simulink model "AMCLIB_FW_BAM"  (Simulink 9.3)
settings: Solver=VariableStepAuto  StartTime=0.0  StopTime=10.0  RelTol=1e-3
settings Model: Creator=nxa18952  LastModifiedBy=nxa18952
settings DataIOCC: SaveFormat=Dataset  SignalLoggingSaveFormat=Dataset  ReturnWorkspaceOutputs=on
settings OptimizationCC: LifeSpan=auto
settings DebuggingCC: UnderspecifiedInitializationDetection=Simplified  MergeDetectMultiDrivingBlocksExec=error  FcnCallInpInsideContextMsg=error  SFUnexpectedBacktrackingDiag=error  SFNoUnconditionalDefaultTransitionDiag=error  SFExecutionAtInitializationDiag=warning  ArithmeticOperatorsInVariantConditions=error
settings HardwareCC: ProdBitPerPointer=64  ProdBitPerSizeT=64  ProdBitPerPtrDiffT=64  ProdLargestAtomicFloat=Float  ProdIntDivRoundTo=Zero  ProdEndianess=LittleEndian  ProdWordSize=64  ProdHWDeviceType=Intel->x86-64 (Windows64)
settings ModelReferenceCC: PropagateSignalLabelsOutOfModel=on
settings SFSimCC: SimUseLocalCustomCode=on
settings RTWCC: RTWUseLocalCustomCode=on
settings CodeAppCC: StateflowObjectComments=off
settings GRTTargetCC: TargetLangStandard=C99 (ISO)  CombineOutputUpdateFcns=on  GRTInterface=off
settings ConfigComp: CovMetricSettings=dwe  CovHtmlReporting=off  CovSaveCumulativeToWorkspaceVar=off  CovSaveSingleToWorkspaceVar=off  CovExternalEMLEnable=on

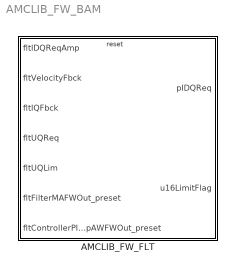
== system AMCLIB_FW_BAM ==
  AMCLIB_FW_FLT : Subsystem  TreatAsAtomicUnit=on  mask(AMCLIB_FW_FLT){showStates=Hide (faster execution), resetStatesEnable=Pre-set according to the first set of inputs after reset, showDebugOutputs=Hide, fltUmaxDivImax=0, fltLambda=0, fltPropGain=0, fltIntegGain=0, fltLowerLimit=0, fltUpperLimit=0}
      mask prompts: showStates "Show internal states"; resetStatesEnable "Internal state after reset"; showDebugOutputs "Show debugging outputs"; fltUmaxDivImax "fltUmaxDivImax (Maximal coil voltage divided by the maximal coil current)"; fltLambda "fltLambda (GDFLIB_FilterMA - smoothing factor)"; fltPropGain "fltPropGain (GFLIB_ControllerPIpAW - proportional gain)"; fltIntegGain "fltIntegGain (GFLIB_ControllerPIpAW - integral gain)"; fltLowerLimit "fltLowerLimit (GFLIB_ControllerPIpAW - lower limit)"; fltUpperLimit "fltUpperLimit (GFLIB_ControllerPIpAW - upper limit)"
      mask help: Field Weakening controller for the PMSM field-oriented control algorithm in single precision floating-point implementation. This block supports re-initialization of the internal state during simulation. If the block is reset, the output of the MA filter and PI controller will be aligned with the inputs fltFilterMAFWOut_preset and fltControllerPIpAWFWOut_preset. Refer to the AMMCLIB User's Guide for further details.
      mask init:
      | if ~evalin('base','exist(''tS8'',''var'')')
      |   if (2 ~= exist('SWLIBS_Typedefs.mat','file'))
      |       error('File SWLIBS_Typedefs.mat is not on the Matlab path. Please add the AMMCLIB "bam" folder in the Matlab Search Path.');
      |   else
      |       evalin('base', 'load(''SWLIBS_Typedefs.mat'')');
      |   end
      | end
      | if showStates == 1
      |     % hidden state variables
      |     if strcmp(get_param([gcb '/fltUmaxDivImax'], 'BlockType'), 'Inport')
      |         posblk = get_param(gcb, 'Position');
      | 
      |         pos = get_param(    [gcb, '/fltUmaxDivImax'], 'Position');
      |         orient = get_param( [gcb, '/fltUmaxDivImax'], 'Orientation');
      |         delete_block(       [gcb, '/fltUmaxDivImax']);
      |         add_block('built-in/Ground', [gcb, '/fltUmaxDivImax'], 'Position', pos, 'Orientation', orient);
      | 
      |         pos = get_param(    [gcb, '/fltLambda'], 'Position');
      |         orient = get_param( [gcb, '/fltLambda'], 'Orientation');
      |         delete_block(       [gcb, '/fltLambda']);
      |         add_block('built-in/Ground', [gcb, '/fltLambda'], 'Position', pos, 'Orientation', orient);
      | 
      |         pos = get_param(    [gcb, '/fltPropGain'], 'Position');
      |         orient = get_param( [gcb, '/fltPropGain'], 'Orientation');
      |         delete_block(       [gcb, '/fltPropGain']);
      |         add_block('built-in/Ground', [gcb, '/fltPropGain'], 'Position', pos, 'Orientation', orient);
      | 
      |         pos = get_param(    [gcb, '/fltIntegGain'], 'Position');
      |         orient = get_param( [gcb, '/fltIntegGain'], 'Orientation');
      |         delete_block(       [gcb, '/fltIntegGain']);
      |         add_block('built-in/Ground', [gcb, '/fltIntegGain'], 'Position', pos, 'Orientation', orient);
      | 
      |         pos = get_param(    [gcb, '/fltLowerLimit'], 'Position');
      |         orient = get_param( [gcb, '/fltLowerLimit'], 'Orientation');
      |         delete_block(       [gcb, '/fltLowerLimit']);
      |         add_block('built-in/Ground', [gcb, '/fltLowerLimit'], 'Position', pos, 'Orientation', orient);
      | 
      |         pos = get_param(    [gcb, '/fltUpperLimit'], 'Position');
      |         orient = get_param( [gcb, '/fltUpperLimit'], 'Orientation');
      |         delete_block(       [gcb, '/fltUpperLimit']);
      |         add_block('built-in/Ground', [gcb, '/fltUpperLimit'], 'Position', pos, 'Orientation', orient);
      | 
      |         pos = get_param(    [gcb, '/fltIQReqK_1'], 'Position');
      |         orient = get_param( [gcb, '/fltIQReqK_1'], 'Orientation');
      |         delete_block(       [gcb, '/fltIQReqK_1']);
      |         add_block('built-in/Ground', [gcb, '/fltIQReqK_1'], 'Position', pos, 'Orientation', orient);
      | 
      |         pos = get_param(    [gcb, '/fltAcc'], 'Position');
      |         orient = get_param( [gcb, '/fltAcc'], 'Orientation');
      |         delete_block(       [gcb, '/fltAcc']);
      |         add_block('built-in/Ground', [gcb, '/fltAcc'], 'Position', pos, 'Orientation', orient);
      | 
      |         pos = get_param(    [gcb, '/fltIntegPartK_1'], 'Position');
      |         orient = get_param( [gcb, '/fltIntegPartK_1'], 'Orientation');
      |         delete_block(       [gcb, '/fltIntegPartK_1']);
      |         add_block('built-in/Ground', [gcb, '/fltIntegPartK_1'], 'Position', pos, 'Orientation', orient);
      | 
      |         pos = get_param(    [gcb, '/fltInK_1'], 'Position');
      |         orient = get_param( [gcb, '/fltInK_1'], 'Orientation');
      |         delete_block(       [gcb, '/fltInK_1']);
      |         add_block('built-in/Ground', [gcb, '/fltInK_1'], 'Position', pos, 'Orientation', orient);
      | 
      | 
      |         pos = get_param(    [gcb '/fltAcc_Out'], 'Position');
      |         orient = get_param( [gcb '/fltAcc_Out'], 'Orientation');
      |         delete_block(       [gcb '/fltAcc_Out']);
      |         add_block('built-in/Terminator', [gcb '/fltAcc_Out'], 'Position', pos, 'Orientation', orient);
      | 
      |         pos = get_param(    [gcb '/fltIntegPartK_1_Out'], 'Position');
      |         orient = get_param( [gcb '/fltIntegPartK_1_Out'], 'Orientation');
      |         delete_block(       [gcb '/fltIntegPartK_1_Out']);
      |         add_block('built-in/Terminator', [gcb '/fltIntegPartK_1_Out'], 'Position', pos, 'Orientation', orient);
      | 
      |         pos = get_param(    [gcb '/fltInK_1_Out'], 'Position');
      |         orient = get_param( [gcb '/fltInK_1_Out'], 'Orientation');
      |         delete_block(       [gcb '/fltInK_1_Out']);
      |         add_block('built-in/Terminator', [gcb '/fltInK_1_Out'], 'Position', pos, 'Orientation', orient);
      | 
      | 
      |         if strcmp(get_param([gcb '/fltIQErrSign'], 'BlockType'), 'Outport')
      |             pos = get_param(    [gcb '/fltIQErrSign'], 'Position');
      |             orient = get_param( [gcb '/fltIQErrSign'], 'Orientation');
      |             delete_block(       [gcb '/fltIQErrSign']);
      |             add_block('built-in/Terminator', [gcb '/fltIQErrSign'], 'Position', pos, 'Orientation', orient);
      | 
      |             pos = get_param(    [gcb '/fltIQErr'], 'Position');
      |             orient = get_param( [gcb '/fltIQErr'], 'Orientation');
      |             delete_block(       [gcb '/fltIQErr']);
      |             add_block('built-in/Terminator', [gcb '/fltIQErr'], 'Position', pos, 'Orientation', orient);
      | 
      |             pos = get_param(    [gcb '/fltFWErr'], 'Position');
      |             orient = get_param( [gcb '/fltFWErr'], 'Orientation');
      |             delete_block(       [gcb '/fltFWErr']);
      |             add_block('built-in/Terminator', [gcb '/fltFWErr'], 'Position', pos, 'Orientation', orient);
      | 
      |             pos = get_param(    [gcb '/fltUQErr'], 'Position');
      |             orient = get_param( [gcb '/fltUQErr'], 'Orientation');
      |             delete_block(       [gcb '/fltUQErr']);
      |             add_block('built-in/Terminator', [gcb '/fltUQErr'], 'Position', pos, 'Orientation', orient);
      | 
      |             pos = get_param(    [gcb '/fltFWErrFilt'], 'Position');
      |             orient = get_param( [gcb '/fltFWErrFilt'], 'Orientation');
      |             delete_block(       [gcb '/fltFWErrFilt']);
      |             add_block('built-in/Terminator', [gcb '/fltFWErrFilt'], 'Position', pos, 'Orientation', orient);
      | 
      |             pos = get_param(    [gcb '/fltFWAngle'], 'Position');
      |             orient = get_param( [gcb '/fltFWAngle'], 'Orientation');
      |             delete_block(       [gcb '/fltFWAngle']);
      |             add_block('built-in/Terminator', [gcb '/fltFWAngle'], 'Position', pos, 'Orientation', orient);
      | 
      |             pos = get_param(    [gcb '/fltFWSin'], 'Position');
      |             orient = get_param( [gcb '/fltFWSin'], 'Orientation');
      |             delete_block(       [gcb '/fltFWSin']);
      |             add_block('built-in/Terminator', [gcb '/fltFWSin'], 'Position', pos, 'Orientation', orient);
      | 
      |             pos = get_param(    [gcb '/fltFWCos'], 'Position');
      |             orient = get_param( [gcb '/fltFWCos'], 'Orientation');
      |             delete_block(       [gcb '/fltFWCos']);
      |             add_block('built-in/Terminator', [gcb '/fltFWCos'], 'Position', pos, 'Orientation', orient);
      | 
      |         end
      | 
      |         set_param([gcb '/fltIDQReqAmp'], 'Port', '1');
      |         set_param([gcb '/fltVelocityFbck'], 'Port', '2');
      |         set_param([gcb '/fltIQFbck'], 'Port', '3');
      |         set_param([gcb '/fltUQReq'], 'Port', '4');
      |         set_param([gcb '/fltUQLim'], 'Port', '5');
      |         set_param([gcb '/fltFilterMAFWOut_preset'], 'Port', '6');
      |         set_param([gcb '/fltControllerPIpAWFWOut_preset'], 'Port', '7');
      | 
      |         set_param([gcb '/pIDQReq'], 'Port', '1');
      |         set_param([gcb '/u16LimitFlag'], 'Port', '2');
      | 
      |         set_param(gcb,'MaskEnables',{'on','on','off','on','on','on','on','on','on'});
      | 
      |         if (posblk(4) - posblk(2)) > 200
      |           height = 200;
      |           set_param(gcb,'Position',[posblk(1), posblk(2), posblk(3), posblk(2)+height])
      |         end
      |     end
      | else
      |     % shown state variables
      |     if strcmp(get_param([gcb '/fltUmaxDivImax'], 'BlockType'), 'Ground')
      |         posblk = get_param(gcb, 'Position');
      | 
      |         pos = get_param(    [gcb, '/fltUmaxDivImax'], 'Position');
      |         orient = get_param( [gcb, '/fltUmaxDivImax'], 'Orientation');
      |         delete_block(       [gcb, '/fltUmaxDivImax']);
      |         add_block('built-in/Inport', [gcb, '/fltUmaxDivImax'], 'Position', pos, 'Orientation', orient, 'OutDataTypeStr', 'single');
      | 
      |         pos = get_param(    [gcb, '/fltLambda'], 'Position');
      |         orient = get_param( [gcb, '/fltLambda'], 'Orientation');
      |         delete_block(       [gcb, '/fltLambda']);
      |         add_block('built-in/Inport', [gcb, '/fltLambda'], 'Position', pos, 'Orientation', orient, 'OutDataTypeStr', 'single');
      | 
      |         pos = get_param(    [gcb, '/fltPropGain'], 'Position');
      |         orient = get_param( [gcb, '/fltPropGain'], 'Orientation');
      |         delete_block(       [gcb, '/fltPropGain']);
      |         add_block('built-in/Inport', [gcb, '/fltPropGain'], 'Position', pos, 'Orientation', orient, 'OutDataTypeStr', 'single');
      | 
      |         pos = get_param(    [gcb, '/fltIntegGain'], 'Position');
      |         orient = get_param( [gcb, '/fltIntegGain'], 'Orientation');
      |         delete_block(       [gcb, '/fltIntegGain']);
      |         add_block('built-in/Inport', [gcb, '/fltIntegGain'], 'Position', pos, 'Orientation', orient, 'OutDataTypeStr', 'single');
      | 
      |         pos = get_param(    [gcb, '/fltLowerLimit'], 'Position');
      |         orient = get_param( [gcb, '/fltLowerLimit'], 'Orientation');
      |         delete_block(       [gcb, '/fltLowerLimit']);
      |         add_block('built-in/Inport', [gcb, '/fltLowerLimit'], 'Position', pos, 'Orientation', orient, 'OutDataTypeStr', 'single');
      | 
      |         pos = get_param(    [gcb, '/fltUpperLimit'], 'Position');
      |         orient = get_param( [gcb, '/fltUpperLimit'], 'Orientation');
      |         delete_block(       [gcb, '/fltUpperLimit']);
      |         add_block('built-in/Inport', [gcb, '/fltUpperLimit'], 'Position', pos, 'Orientation', orient, 'OutDataTypeStr', 'single');
      | 
      |         pos = get_param(    [gcb, '/fltIQReqK_1'], 'Position');
      |         orient = get_param( [gcb, '/fltIQReqK_1'], 'Orientation');
      |         delete_block(       [gcb, '/fltIQReqK_1']);
      |         add_block('built-in/Inport', [gcb, '/fltIQReqK_1'], 'Position', pos, 'Orientation', orient, 'OutDataTypeStr', 'single');
      | 
      |         pos = get_param(    [gcb, '/fltAcc'], 'Position');
      |         orient = get_param( [gcb, '/fltAcc'], 'Orientation');
      |         delete_block(       [gcb, '/fltAcc']);
      |         add_block('built-in/Inport', [gcb, '/fltAcc'], 'Position', pos, 'Orientation', orient, 'OutDataTypeStr', 'single');
      | 
      |         pos = get_param(    [gcb, '/fltIntegPartK_1'], 'Position');
      |         orient = get_param( [gcb, '/fltIntegPartK_1'], 'Orientation');
      |         delete_block(       [gcb, '/fltIntegPartK_1']);
      |         add_block('built-in/Inport', [gcb, '/fltIntegPartK_1'], 'Position', pos, 'Orientation', orient, 'OutDataTypeStr', 'single');
      | 
      |         pos = get_param(    [gcb, '/fltInK_1'], 'Position');
      |         orient = get_param( [gcb, '/fltInK_1'], 'Orientation');
      |         delete_block(       [gcb, '/fltInK_1']);
      |         add_block('built-in/Inport', [gcb, '/fltInK_1'], 'Position', pos, 'Orientation', orient, 'OutDataTypeStr', 'single');
      | 
      | 
      |         pos = get_param(    [gcb '/fltAcc_Out'], 'Position');
      |         orient = get_param( [gcb '/fltAcc_Out'], 'Orientation');
      |         delete_block(       [gcb '/fltAcc_Out']);
      |         add_block('built-in/Outport', [gcb '/fltAcc_Out'], 'Position', pos, 'Orientation', orient);
      | 
      |         pos = get_param(    [gcb '/fltIntegPartK_1_Out'], 'Position');
      |         orient = get_param( [gcb '/fltIntegPartK_1_Out'], 'Orientation');
      |         delete_block(       [gcb '/fltIntegPartK_1_Out']);
      |         add_block('built-in/Outport', [gcb '/fltIntegPartK_1_Out'], 'Position', pos, 'Orientation', orient);
      | 
      |         pos = get_param(    [gcb '/fltInK_1_Out'], 'Position');
      |         orient = get_param( [gcb '/fltInK_1_Out'], 'Orientation');
      |         delete_block(       [gcb '/fltInK_1_Out']);
      |         add_block('built-in/Outport', [gcb '/fltInK_1_Out'], 'Position', pos, 'Orientation', orient);
      | 
      | 
      |         if (showDebugOutputs == 2) && (strcmp(get_param([gcb '/fltIQErrSign'], 'BlockType'), 'Terminator'))
      |             pos = get_param(    [gcb '/fltIQErrSign'], 'Position');
      |             orient = get_param( [gcb '/fltIQErrSign'], 'Orientation');
      |             delete_block(       [gcb '/fltIQErrSign']);
      |             add_block('built-in/Outport', [gcb '/fltIQErrSign'], 'Position', pos, 'Orientation', orient);
      | 
      |             pos = get_param(    [gcb '/fltIQErr'], 'Position');
      |             orient = get_param( [gcb '/fltIQErr'], 'Orientation');
      |             delete_block(       [gcb '/fltIQErr']);
      |             add_block('built-in/Outport', [gcb '/fltIQErr'], 'Position', pos, 'Orientation', orient);
      | 
      |             pos = get_param(    [gcb '/fltFWErr'], 'Position');
      |             orient = get_param( [gcb '/fltFWErr'], 'Orientation');
      |             delete_block(       [gcb '/fltFWErr']);
      |             add_block('built-in/Outport', [gcb '/fltFWErr'], 'Position', pos, 'Orientation', orient);
      | 
      |             pos = get_param(    [gcb '/fltUQErr'], 'Position');
      |             orient = get_param( [gcb '/fltUQErr'], 'Orientation');
      |             delete_block(       [gcb '/fltUQErr']);
      |             add_block('built-in/Outport', [gcb '/fltUQErr'], 'Position', pos, 'Orientation', orient);
      | 
      |             pos = get_param(    [gcb '/fltFWErrFilt'], 'Position');
      |             orient = get_param( [gcb '/fltFWErrFilt'], 'Orientation');
      |             delete_block(       [gcb '/fltFWErrFilt']);
      |             add_block('built-in/Outport', [gcb '/fltFWErrFilt'], 'Position', pos, 'Orientation', orient);
      | 
      |             pos = get_param(    [gcb '/fltFWAngle'], 'Position');
      |             orient = get_param( [gcb '/fltFWAngle'], 'Orientation');
      |             delete_block(       [gcb '/fltFWAngle']);
      |             add_block('built-in/Outport', [gcb '/fltFWAngle'], 'Position', pos, 'Orientation', orient);
      | 
      |             pos = get_param(    [gcb '/fltFWSin'], 'Position');
      |             orient = get_param( [gcb '/fltFWSin'], 'Orientation');
      |             delete_block(       [gcb '/fltFWSin']);
      |             add_block('built-in/Outport', [gcb '/fltFWSin'], 'Position', pos, 'Orientation', orient);
      | 
      |             pos = get_param(    [gcb '/fltFWCos'], 'Position');
      |             orient = get_param( [gcb '/fltFWCos'], 'Orientation');
      |             delete_block(       [gcb '/fltFWCos']);
      |             add_block('built-in/Outport', [gcb '/fltFWCos'], 'Position', pos, 'Orientation', orient);
      | 
      |         end
      | 
      |         set_param([gcb '/fltIDQReqAmp'], 'Port', '1');
      |         set_param([gcb '/fltVelocityFbck'], 'Port', '2');
      |         set_param([gcb '/fltIQFbck'], 'Port', '3');
      |         set_param([gcb '/fltUQReq'], 'Port', '4');
      |         set_param([gcb '/fltUQLim'], 'Port', '5');
      |         set_param([gcb '/fltFilterMAFWOut_preset'], 'Port', '6');
      |         set_param([gcb '/fltControllerPIpAWFWOut_preset'], 'Port', '7');
      |         set_param([gcb '/fltUmaxDivImax'], 'Port', '8');
      |         set_param([gcb '/fltLambda'], 'Port', '9');
      |         set_param([gcb '/fltPropGain'], 'Port', '10');
      |         set_param([gcb '/fltIntegGain'], 'Port', '11');
      |         set_param([gcb '/fltLowerLimit'], 'Port', '12');
      |         set_param([gcb '/fltUpperLimit'], 'Port', '13');
      |         set_param([gcb '/fltIQReqK_1'], 'Port', '14');
      |         set_param([gcb '/fltAcc'], 'Port', '15');
      |         set_param([gcb '/fltIntegPartK_1'], 'Port', '16');
      |         set_param([gcb '/fltInK_1'], 'Port', '17');
      | 
      |         if (showDebugOutputs == 2)
      |             set_param([gcb '/pIDQReq'], 'Port', '1');
      |             set_param([gcb '/u16LimitFlag'], 'Port', '2');
      |             set_param([gcb '/fltIQErrSign'], 'Port', '3');
      |             set_param([gcb '/fltIQErr'], 'Port', '4');
      |             set_param([gcb '/fltFWErr'], 'Port', '5');
      |             set_param([gcb '/fltUQErr'], 'Port', '6');
      |             set_param([gcb '/fltFWErrFilt'], 'Port', '7');
      |             set_param([gcb '/fltFWAngle'], 'Port', '8');
      |             set_param([gcb '/fltFWSin'], 'Port', '9');
      |             set_param([gcb '/fltFWCos'], 'Port', '10');
      |             set_param([gcb '/fltAcc_Out'], 'Port', '11');
      |             set_param([gcb '/fltIntegPartK_1_Out'], 'Port', '12');
      |             set_param([gcb '/fltInK_1_Out'], 'Port', '13');
      |         else
      |             set_param([gcb '/pIDQReq'], 'Port', '1');
      |             set_param([gcb '/u16LimitFlag'], 'Port', '2');
      |             set_param([gcb '/fltAcc_Out'], 'Port', '3');
      |             set_param([gcb '/fltIntegPartK_1_Out'], 'Port', '4');
      |             set_param([gcb '/fltInK_1_Out'], 'Port', '5');
      |         end
      | 
      |         set_param(gcb,'MaskEnables',{'on','on','on','off','off','off','off','off','off'});
      | 
      |         if (posblk(4) - posblk(2)) < 450
      |           height = 450;
      |           set_param(gcb,'Position',[posblk(1), posblk(2), posblk(3), posblk(2)+height])
      |         end
      |     else
      |         if (showDebugOutputs == 2) && (strcmp(get_param([gcb '/fltIQErrSign'], 'BlockType'), 'Terminator'))
      |             % shown debugging outputs
      |             pos = get_param(    [gcb '/fltIQErrSign'], 'Position');
      |             orient = get_param( [gcb '/fltIQErrSign'], 'Orientation');
      |             delete_block(       [gcb '/fltIQErrSign']);
      |             add_block('built-in/Outport', [gcb '/fltIQErrSign'], 'Position', pos, 'Orientation', orient);
      | 
      |             pos = get_param(    [gcb '/fltIQErr'], 'Position');
      |             orient = get_param( [gcb '/fltIQErr'], 'Orientation');
      |             delete_block(       [gcb '/fltIQErr']);
      |             add_block('built-in/Outport', [gcb '/fltIQErr'], 'Position', pos, 'Orientation', orient);
      | 
      |             pos = get_param(    [gcb '/fltFWErr'], 'Position');
      |             orient = get_param( [gcb '/fltFWErr'], 'Orientation');
      |             delete_block(       [gcb '/fltFWErr']);
      |             add_block('built-in/Outport', [gcb '/fltFWErr'], 'Position', pos, 'Orientation', orient);
      | 
      |             pos = get_param(    [gcb '/fltUQErr'], 'Position');
      |             orient = get_param( [gcb '/fltUQErr'], 'Orientation');
      |             delete_block(       [gcb '/fltUQErr']);
      |             add_block('built-in/Outport', [gcb '/fltUQErr'], 'Position', pos, 'Orientation', orient);
      | 
      |             pos = get_param(    [gcb '/fltFWErrFilt'], 'Position');
      |             orient = get_param( [gcb '/fltFWErrFilt'], 'Orientation');
      |             delete_block(       [gcb '/fltFWErrFilt']);
      |             add_block('built-in/Outport', [gcb '/fltFWErrFilt'], 'Position', pos, 'Orientation', orient);
      | 
      |             pos = get_param(    [gcb '/fltFWAngle'], 'Position');
      |             orient = get_param( [gcb '/fltFWAngle'], 'Orientation');
      |             delete_block(       [gcb '/fltFWAngle']);
      |             add_block('built-in/Outport', [gcb '/fltFWAngle'], 'Position', pos, 'Orientation', orient);
      | 
      |             pos = get_param(    [gcb '/fltFWSin'], 'Position');
      |             orient = get_param( [gcb '/fltFWSin'], 'Orientation');
      |             delete_block(       [gcb '/fltFWSin']);
      |             add_block('built-in/Outport', [gcb '/fltFWSin'], 'Position', pos, 'Orientation', orient);
      | 
      |             pos = get_param(    [gcb '/fltFWCos'], 'Position');
      |             orient = get_param( [gcb '/fltFWCos'], 'Orientation');
      |             delete_block(       [gcb '/fltFWCos']);
      |             add_block('built-in/Outport', [gcb '/fltFWCos'], 'Position', pos, 'Orientation', orient);
      | 
      |             set_param([gcb '/pIDQReq'], 'Port', '1');
      |             set_param([gcb '/u16LimitFlag'], 'Port', '2');
      |             set_param([gcb '/fltIQErrSign'], 'Port', '3');
      |             set_param([gcb '/fltIQErr'], 'Port', '4');
      |             set_param([gcb '/fltFWErr'], 'Port', '5');
      |             set_param([gcb '/fltUQErr'], 'Port', '6');
      |             set_param([gcb '/fltFWErrFilt'], 'Port', '7');
      |             set_param([gcb '/fltFWAngle'], 'Port', '8');
      |             set_param([gcb '/fltFWSin'], 'Port', '9');
      |             set_param([gcb '/fltFWCos'], 'Port', '10');
      |             set_param([gcb '/fltAcc_Out'], 'Port', '11');
      |             set_param([gcb '/fltIntegPartK_1_Out'], 'Port', '12');
      |             set_param([gcb '/fltInK_1_Out'], 'Port', '13');
      |         elseif (showDebugOutputs == 1) && (strcmp(get_param([gcb '/fltIQErrSign'], 'BlockType'), 'Outport'))
      |             % hidden debugging outputs
      |             pos = get_param(    [gcb '/fltIQErrSign'], 'Position');
      |             orient = get_param( [gcb '/fltIQErrSign'], 'Orientation');
      |             delete_block(       [gcb '/fltIQErrSign']);
      |             add_block('built-in/Terminator', [gcb '/fltIQErrSign'], 'Position', pos, 'Orientation', orient);
      | 
      |             pos = get_param(    [gcb '/fltIQErr'], 'Position');
      |             orient = get_param( [gcb '/fltIQErr'], 'Orientation');
      |             delete_block(       [gcb '/fltIQErr']);
      |             add_block('built-in/Terminator', [gcb '/fltIQErr'], 'Position', pos, 'Orientation', orient);
      | 
      |             pos = get_param(    [gcb '/fltFWErr'], 'Position');
      |             orient = get_param( [gcb '/fltFWErr'], 'Orientation');
      |             delete_block(       [gcb '/fltFWErr']);
      |             add_block('built-in/Terminator', [gcb '/fltFWErr'], 'Position', pos, 'Orientation', orient);
      | 
      |             pos = get_param(    [gcb '/fltUQErr'], 'Position');
      |             orient = get_param( [gcb '/fltUQErr'], 'Orientation');
      |             delete_block(       [gcb '/fltUQErr']);
      |             add_block('built-in/Terminator', [gcb '/fltUQErr'], 'Position', pos, 'Orientation', orient);
      | 
      |             pos = get_param(    [gcb '/fltFWErrFilt'], 'Position');
      |             orient = get_param( [gcb '/fltFWErrFilt'], 'Orientation');
      |             delete_block(       [gcb '/fltFWErrFilt']);
      |             add_block('built-in/Terminator', [gcb '/fltFWErrFilt'], 'Position', pos, 'Orientation', orient);
      | 
      |             pos = get_param(    [gcb '/fltFWAngle'], 'Position');
      |             orient = get_param( [gcb '/fltFWAngle'], 'Orientation');
      |             delete_block(       [gcb '/fltFWAngle']);
      |             add_block('built-in/Terminator', [gcb '/fltFWAngle'], 'Position', pos, 'Orientation', orient);
      | 
      |             pos = get_param(    [gcb '/fltFWSin'], 'Position');
      |             orient = get_param( [gcb '/fltFWSin'], 'Orientation');
      |             delete_block(       [gcb '/fltFWSin']);
      |             add_block('built-in/Terminator', [gcb '/fltFWSin'], 'Position', pos, 'Orientation', orient);
      | 
      |             pos = get_param(    [gcb '/fltFWCos'], 'Position');
      |             orient = get_param( [gcb '/fltFWCos'], 'Orientation');
      |             delete_block(       [gcb '/fltFWCos']);
      |             add_block('built-in/Terminator', [gcb '/fltFWCos'], 'Position', pos, 'Orientation', orient);
      | 
      |             set_param([gcb '/pIDQReq'], 'Port', '1');
      |             set_param([gcb '/u16LimitFlag'], 'Port', '2');
      |             set_param([gcb '/fltAcc_Out'], 'Port', '3');
      |             set_param([gcb '/fltIntegPartK_1_Out'], 'Port', '4');
      |             set_param([gcb '/fltInK_1_Out'], 'Port', '5');
      |         end
      |     end
      | end
      settings: RTWSystemCode=Inline
      mask TypeOptions showStates: Hide (faster execution) | Show (allows debugging; connect feedback loops manually)
      mask Callback showStates:
      | maskStr = get_param(gcb,'showStates');
      | if strcmp(maskStr,'Hide (faster execution)'),
      |     set_param(gcb,'MaskEnables',{'on','on','off','on','on','on','on','on','on'});
      | else
      |     set_param(gcb,'MaskEnables',{'on','on','on','off','off','off','off','off','off'});
      | end
      mask TypeOptions resetStatesEnable: Pre-set according to the first set of inputs after reset | Clear to zero
      mask TypeOptions showDebugOutputs: Hide | Show
      mask Display:
      | color('black');
      | pos = get_param(gcb, 'Position');
      | width = pos(3) - pos(1);
      | height = pos(4) - pos(2);
      | tX=width/2;
      | tY=height - 25;
      | color('black');
      | text(tX,tY, 'AMCLIB_FW_FLT', 'horizontalAlignment', 'center');
      | if showStates == 2
      |   color('red');
      |   text(tX,tY - 20, ['debugging mode' char(13) char(10) '(limited performance)'], 'horizontalAlignment', 'center');
      | end

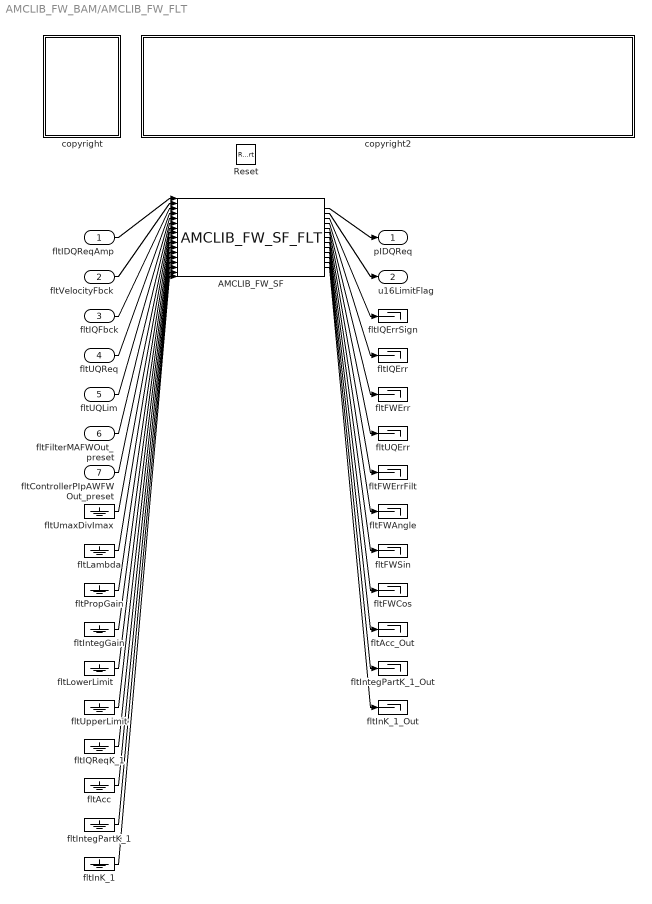
== system AMCLIB_FW_BAM/AMCLIB_FW_FLT ==
  fltIDQReqAmp : Inport  OutDataTypeStr=single
  fltVelocityFbck : Inport  Port=2  OutDataTypeStr=single
  fltIQFbck : Inport  Port=3  OutDataTypeStr=single
  fltUQReq : Inport  Port=4  OutDataTypeStr=single
  fltUQLim : Inport  Port=5  OutDataTypeStr=single
  fltFilterMAFWOut_preset : Inport  Port=6  OutDataTypeStr=single
  fltControllerPIpAWFWOut_preset : Inport  Port=7  OutDataTypeStr=single
  Reset : ResetPort  DisableCoverage=on
  AMCLIB_FW_SF : S-Function  FunctionName=AMCLIB_FW_SF_FLT  Parameters=showStates,resetStatesEnable,showDebugOutputs,fltUmaxDivImax,fltLambda,fltPropGain,fltIntegGain,fltLowerLimit,fltUpperLimit  SFunctionDeploymentMode=off  EnableBusSupport=off
  copyright : Subsystem
      mask Display: text(10,90,'FILE:');text(10,75,'DESRIPTION:');text(10,60,'COPYRIGHT:');text(10,45,'VERSION:');text(10,30,'DATE:')
  copyright2 : Subsystem
      mask Display: text(10,90,'AMCLIB_FW_BAM_FLT.mdl');text(10,75,'PMSM Field Weakening Controller');text(10,60,'NXP 2020');text(10,45,'1.0');text(10,30,'28-Mar-2020');
  fltAcc : Ground
  fltAcc_Out : Terminator
  fltFWAngle : Terminator
  fltFWCos : Terminator
  fltFWErr : Terminator
  fltFWErrFilt : Terminator
  fltFWSin : Terminator
  fltIQErr : Terminator
  fltIQErrSign : Terminator
  fltIQReqK_1 : Ground
  fltInK_1 : Ground
  fltInK_1_Out : Terminator
  fltIntegGain : Ground
  fltIntegPartK_1 : Ground
  fltIntegPartK_1_Out : Terminator
  fltLambda : Ground
  fltLowerLimit : Ground
  fltPropGain : Ground
  fltUQErr : Terminator
  fltUmaxDivImax : Ground
  fltUpperLimit : Ground
  pIDQReq : Outport
  u16LimitFlag : Outport  Port=2
  wires:
  fltIDQReqAmp/1 -> AMCLIB_FW_SF/1
  fltVelocityFbck/1 -> AMCLIB_FW_SF/2
  fltIQFbck/1 -> AMCLIB_FW_SF/3
  fltUQReq/1 -> AMCLIB_FW_SF/4
  fltUQLim/1 -> AMCLIB_FW_SF/5
  fltFilterMAFWOut_preset/1 -> AMCLIB_FW_SF/6
  fltControllerPIpAWFWOut_preset/1 -> AMCLIB_FW_SF/7
  fltUmaxDivImax/1 -> AMCLIB_FW_SF/8
  fltLambda/1 -> AMCLIB_FW_SF/9
  fltPropGain/1 -> AMCLIB_FW_SF/10
  fltIntegGain/1 -> AMCLIB_FW_SF/11
  fltLowerLimit/1 -> AMCLIB_FW_SF/12
  fltUpperLimit/1 -> AMCLIB_FW_SF/13
  fltIQReqK_1/1 -> AMCLIB_FW_SF/14
  fltAcc/1 -> AMCLIB_FW_SF/15
  fltIntegPartK_1/1 -> AMCLIB_FW_SF/16
  fltInK_1/1 -> AMCLIB_FW_SF/17
  AMCLIB_FW_SF/1 -> pIDQReq/1
  AMCLIB_FW_SF/2 -> u16LimitFlag/1
  AMCLIB_FW_SF/3 -> fltIQErrSign/1
  AMCLIB_FW_SF/4 -> fltIQErr/1
  AMCLIB_FW_SF/5 -> fltFWErr/1
  AMCLIB_FW_SF/6 -> fltUQErr/1
  AMCLIB_FW_SF/7 -> fltFWErrFilt/1
  AMCLIB_FW_SF/8 -> fltFWAngle/1
  AMCLIB_FW_SF/9 -> fltFWSin/1
  AMCLIB_FW_SF/10 -> fltFWCos/1
  AMCLIB_FW_SF/11 -> fltAcc_Out/1
  AMCLIB_FW_SF/12 -> fltIntegPartK_1_Out/1
  AMCLIB_FW_SF/13 -> fltInK_1_Out/1

== system AMCLIB_FW_BAM/AMCLIB_FW_FLT/copyright ==

== system AMCLIB_FW_BAM/AMCLIB_FW_FLT/copyright2 ==
